simulink model "sl1"  (Simulink 7.2)
settings: Solver=ode3  StartTime=0.0  StopTime=50  FixedStep=0.002  RelTol=1e-3
settings Model: Creator=controle  LastModifiedBy=controle  ExtModeTrigDuration=5000
settings SolverCC: PositivePriorityOrder=on
settings RTWCC: SystemTargetFile=quarc_windows.tlc  TemplateMakefile=quarc_default_tmf  Description=QUARC Win32 Target  ProcessScript=quarc_windows_make_rtw_hook
settings STFCustomTargetCC: TargetPreCompLibLocation=C:\DOCUME~1\ALLUSE~1\DADOSD~1\QUARC\lib\2008b\windows\release  SystemTargetFile=quarc_windows.tlc
settings GRTTargetCC: TargetPreCompLibLocation=C:\DOCUME~1\ALLUSE~1\DADOSD~1\QUARC\lib\2008b\windows\release  CompOptLevelCompliant=off  MatFileLogging=off  ExtMode=on  ExtModeMexFile=quarc_comm

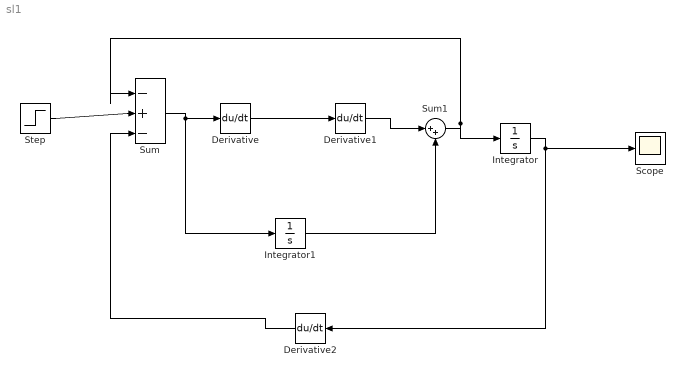
== system sl1 ==
  Derivative : Derivative
  Derivative1 : Derivative
  Derivative2 : Derivative  Orientation=left
  Integrator : Integrator
  Integrator1 : Integrator
  Scope : Scope
      settings: YMin=-3.25e+051  YMax=1e+051
  Step : Step  SampleTime=0
  Sum : Sum  Inputs=|-+-  OutDataType=sfix(16)  OutScaling=2^0
  Sum1 : Sum  Inputs=|++  OutDataType=sfix(16)  OutScaling=2^0
  wires:
  Step/1 -> Sum/2
  Sum/1 -> Derivative/1, Integrator1/1
  Derivative/1 -> Derivative1/1
  Derivative1/1 -> Sum1/1
  Sum1/1 -> Integrator/1, Sum/1
  Integrator1/1 -> Sum1/2
  Integrator/1 -> Derivative2/1, Scope/1
  Derivative2/1 -> Sum/3
